simulink model "simulation_model"  (R2022a)
settings: Solver=VariableStepAuto  StartTime=0.0  StopTime=500  MaxStep=0.1  RelTol=1e-3
values from neighbouring files (symbols this model uses):
  gamma_pb = deg2rad(24.6)    [example_m.m]
  psi0 = atan(yc/xc)    [example_m.m]
  xc = 410    [example_m.m]
  yc = -120    [example_m.m]
undefined symbols (not defined in the file or in its folder): sigbuilder_block
libraries: simulink_extras x4, simulink x1
(part 3 of 3)

== matlab function simulation_model/Missile dynamics model/Forces acting on the object /Aerodynamic Force ==
  data: C_X0 input; R output; rho input; C_Na_ster input; C_Na_kadl input; alfa_t input; C_Xa2 input; U input; V input; W input; alfa input; beta input; delta_w input; delta_k input
%% function which calculates Components of the aerodynamic force
% 
% Inputs:
% C_X0 - Axial force coefficient (\alpha_t = 0)
% rho - air density [kg/m^3]
% C_Na_ster - Derivative of normal force coefficient after sin\alpha for fins
% C_Na_kadl - Derivative of normal force coefficient after sin\alpha for monocoque
% alfa_t - total angle of attack [rad]
% C_Xa2 - Derivative of axial force coefficient after sin^2\alpha_t
% U - velocity about x body axis [m/s]
% V - velocity about y body axis [m/s]
% W - velocity about z body axis [m/s]
% alfa - angle of attack [rad]
% beta - angle of sideslip [rad] 
% delta_w deflection of fins in axis Z [rad]
% delta_k - deflection of fins in axis Y [rad]
%
% Outputs:
% R - Aerodynamic force [N]


function R = fcn(C_X0, rho, C_Na_ster, C_Na_kadl, alfa_t, C_Xa2, U, V, W, alfa, beta, delta_w, delta_k)
R = zeros(3,1);

% calculate cross-sectional area
S = pi*(0.92/2)^2;

% calculate the absolute value of velocity
Vaer_bezwzgl = sqrt(U^2 + V^2 + W^2);

% calculate axial force
P_x = (C_X0 + C_Xa2*sin(alfa_t)^2)*0.5*rho*Vaer_bezwzgl^2*S;
P_x_x = -P_x;

% calculate normal force  and sideforce coefficients
C_N_y = C_Na_kadl*sin(beta) + C_Na_ster*sin(beta+delta_k);
C_N_z = C_Na_kadl*cos(beta)*sin(alfa) + C_Na_ster*cos(beta)*sin(alfa+delta_w);

% calculate normal force and sideforce
P_N_y = -C_N_y*0.5*rho*Vaer_bezwzgl^2*S;
P_N_z = -C_N_z*0.5*rho*Vaer_bezwzgl^2*S;

R = [P_x_x; P_N_y; P_N_z];
